simulink model "untitled"  (R2022b)
settings: Solver=VariableStepAuto  StartTime=0.0  StopTime=10.0  RelTol=1e-3
values from neighbouring files (symbols this model uses):
  Ad = plant_d.A    [CartPole.m]
  Bd = plant_d.B    [CartPole.m]
  Cd = plant_d.C    [CartPole.m]
  Dd = plant_d.D    [CartPole.m]
  ref = [0; 0; 0; 0]    [CartPole.m]
  Ts = 0.02    [CartPole.m]
  x0 = [0; 0; theta0; 0]    [CartPole.m]
libraries: mpclib x1
settings Model: Creator=TM  LastModifiedBy=TM

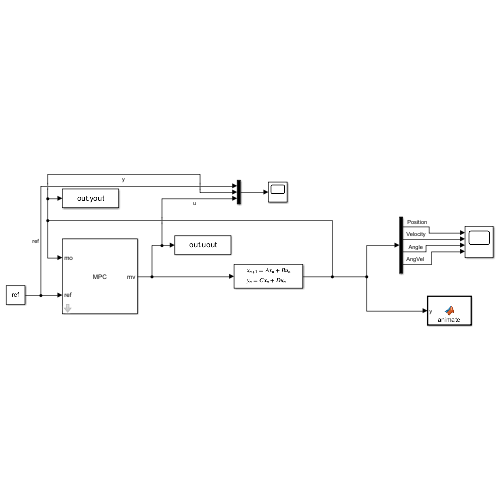
[thumbnail: Simulink's stored preview of the top-level diagram]
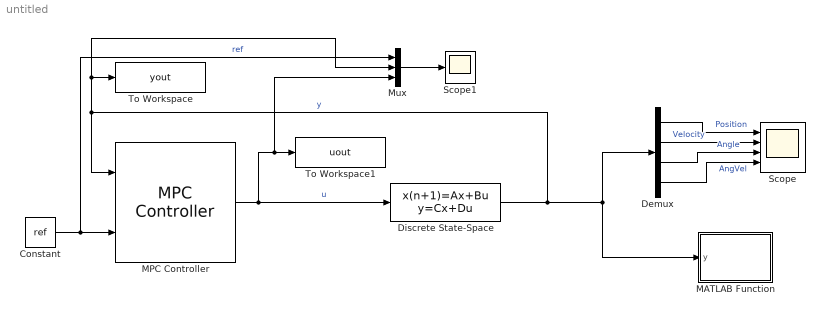
== system untitled ==
  Constant : Constant  Value=ref
  Demux : Demux
  Discrete State-Space : DiscreteStateSpace  A=Ad  B=Bd  C=Cd  D=Dd  InitialCondition=x0  SampleTime=Ts
  MATLAB Function : MATLAB Function  TreatAsAtomicUnit=on
  MPC Controller : mpclib/MPC Controller  SCDEnableBlockLinearizationSpecification=on  mpcobj=mpcobj  is_multiple=0  enable_value=0  return_u0=off  updateMPCinCallerWorkspace=on  md_inport=off  mv_inport=off  uref_inport=off  return_cost=off  return_mvseq=off  return_qpstatus=off  return_xseq=off  return_state=off  return_ovseq=off  state_inport=off  umin_inport=off  umax_inport=off  ymin_inport=off  ymax_inport=off  cc_inport=off  ywt_inport=off  uwt_inport=off  duwt_inport=off  rhoeps_inport=off  pm_inport=off  MaximumP=10  HorizonChoice=FixedHorizon  n_ts=0.02  n_p=50  n_mv=1  n_md=0  n_ud=0  n_mo=4  n_uo=0  BlockDataType=double  SampleTimeInherited=off  switch_inport=off
  Mux : Mux  Inputs=3
  Scope : Scope  NumInputPorts=4
  Scope1 : Scope
  To Workspace : ToWorkspace  VariableName=yout  SaveFormat=Timeseries  SampleTime=-1
  To Workspace1 : ToWorkspace  VariableName=uout  SaveFormat=Timeseries  SampleTime=-1
  wires:
  Constant/1 -> Mux/1, MPC Controller/2  "ref"
  MPC Controller/1 -> Discrete State-Space/1, Mux/3, To Workspace1/1  "u"
  Discrete State-Space/1 -> Mux/2, To Workspace/1, MPC Controller/1, MATLAB Function/1(y), Demux/1  "y"
  Demux/1 -> Scope/1  "Position"
  Demux/2 -> Scope/2  "Velocity"
  Demux/3 -> Scope/3  "Angle"
  Demux/4 -> Scope/4  "AngVel"
  Mux/1 -> Scope1/1

== matlab function untitled/MATLAB Function ==
  data: y input
function animate(y)
coder.extrinsic('cartpole_sim');
x = y(1);
theta = y(3);
cartpole_sim(x, theta);
